simulink model "running_contact_state_machine"  (R2015a)
settings: Solver=ode45  StartTime=0.0  StopTime=10.0  RelTol=1e-3
undefined symbols (not defined in the file): body_weight, contact_threshold, g, loaded_threshold, sample_time, t_flight
libraries: simulink x1
settings Model: Creator=wmartin  LastModifiedBy=wmartin

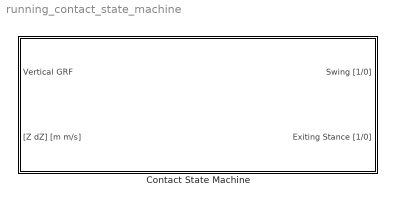
== system running_contact_state_machine ==
  Contact State Machine : Subsystem

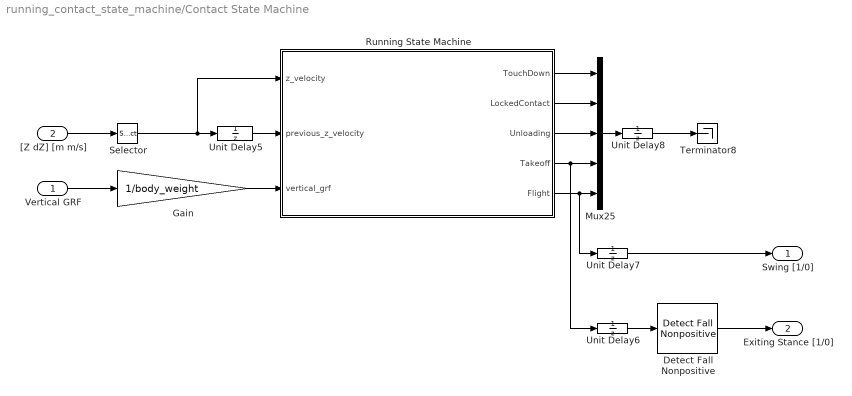
== system running_contact_state_machine/Contact State Machine ==
  Vertical GRF : Inport
  "[Z dZ] [m m/s]" : Inport  Port=2
  Detect Fall Nonpositive : simulink/Logic and Bit Operations/Detect Fall Nonpositive  vinit=1  InputProcessing=Inherited  OutDataTypeStr=boolean
  Gain : Gain  Gain=1/body_weight
  Mux25 : Mux  Inputs=5
  Running State Machine : State Transition Table  TreatAsAtomicUnit=on
  Selector : Selector  InputPortWidth=2  Indices=[2]
  Terminator8 : Terminator
  Unit Delay5 : UnitDelay  SampleTime=-1
  Unit Delay6 : UnitDelay  SampleTime=sample_time
  Unit Delay7 : UnitDelay  InitialCondition=1  SampleTime=sample_time
  Unit Delay8 : UnitDelay  SampleTime=sample_time
  Swing [1/0] : Outport
  Exiting Stance [1/0] : Outport  Port=2
  wires:
  "[Z dZ] [m m/s]"/1 -> Selector/1
  Running State Machine/1(" TouchDown") -> Mux25/1
  Running State Machine/2(" LockedContact") -> Mux25/2
  Running State Machine/3(" Unloading") -> Mux25/3
  Mux25/1 -> Unit Delay8/1
  Running State Machine/5(" Flight") -> Unit Delay7/1, Mux25/5
  Unit Delay5/1 -> Running State Machine/2(previous_z_velocity)
  Gain/1 -> Running State Machine/3(vertical_grf)
  Selector/1 -> Unit Delay5/1, Running State Machine/1(z_velocity)
  Unit Delay8/1 -> Terminator8/1
  Running State Machine/4(" Takeoff") -> Mux25/4, Unit Delay6/1
  Unit Delay6/1 -> Detect Fall Nonpositive/1
  Unit Delay7/1 -> Swing [1/0]/1
  Detect Fall Nonpositive/1 -> Exiting Stance [1/0]/1
  Vertical GRF/1 -> Gain/1

== stateflow chart running_contact_state_machine/Contact State Machine/Running State Machine ==
  state TouchDown
  state LockedContact
  state Unloading
  state Takeoff
  state Flight
  (junction 91) -> TouchDown
  TouchDown -> (junction 130) [order 2] : [vertical_grf < contact_threshold]
  (junction 93) -> (junction 91)
  (junction 130) -> (junction 128)
  TouchDown -> LockedContact [order 1] : [vertical_grf > loaded_threshold]
  (junction 115) -> LockedContact
  (junction 118) -> (junction 115)
  LockedContact -> Unloading : [z_velocity >= 0 && previous_z_velocity < 0]
  Unloading -> LockedContact [order 2] : [vertical_grf > loaded_threshold && z_velocity < 0]
  (junction 122) -> (junction 118)
  Unloading -> Takeoff [order 1] : [vertical_grf < contact_threshold]
  Takeoff -> Flight : after(t_flight,sec)
  (default) -> Flight
  Flight -> (junction 93) : [vertical_grf > contact_threshold]
  (junction 128) -> Flight
  data: z_velocity input; previous_z_velocity input; vertical_grf input; t_flight parameter; g parameter; contact_threshold parameter; loaded_threshold parameter; TouchDown output boolean; LockedContact output boolean; Unloading output boolean; Takeoff output boolean; Flight output boolean
